simulink model "M2C_IM_CL_V1_NCADMM_Sim"  (R2023a)
settings: Solver=ode4  StartTime=0.0  StopTime=t_sim  FixedStep=tsim  RelTol=1e-3
model workspace (MAT data in the model file):
  global_can_baud_rate = '1000000'
  global_ip_addresses = {'', '', '', ''}
values from neighbouring files (symbols this model uses):
  A = [1 1 1 0 0 0 ... (first row only)    [M2C_init.m]    (also in MMCC_Sim_Script_BCD_activeset.m = -[1 0 0 1 0 0 1 0 0; 0 1 0 0 1 0 0 1 0; 0 0 1 0 0 1 0 0 1; -; MMCC_Sim_Script_BCD_activeset_LH.m = -[1 0 0 1 0 0 1 0 0; 0 1 0 0 1 0 0 1 0; 0 0 1 0 0 1 0 0 1; -)
  A11 = -(1/tau_sig)*eye(2)    [M2C_init.m]
  A21 = (Lm/tau_r)*eye(2)    [M2C_init.m]
  A_admm = zeros(2*Np, Np)    [M2C_init.m]
  A_cc = [1 0 ... (first row only)    [M2C_init.m]
  b_admm_1 = imax_admm*ones(2*Np,1)    [M2C_init.m]
  b_cc = Vmax_cc*ones(4,1)    [M2C_init.m]
  c_admm = -imax_admm*ones(Np,1)    [M2C_init.m]
  C_obs = [eye(2) zeros(2)]    [M2C_init.m]
  C_sm = 987e-6    (= 0.000987)    [M2C_init.m]
  G_cc = [1 1 ... (first row only)    [M2C_init.m]
  J_imag = [0 -1 ... (first row only)    [M2C_init.m]
  K_obsm = K_obs2'    [M2C_init.m]
  K_obsp = K_obs1'    [M2C_init.m]
  kr = Lm/Lr    (= 0.989061842659)    [M2C_init.m]
  L = 5e-3    (= 0.005)    [M2C_init.m]    (also in MMCC_Sim_Script_BCD_activeset.m = 0.02; MMCC_Sim_Script_BCD_activeset_LH.m = 0.02)
  Lsigmar = 2.6e-3    (= 0.0026)    [M2C_init.m]
  Lsigmas = 2.6e-3    (= 0.0026)    [M2C_init.m]
  N = [1/sqrt(3) 0;-1/(2*sqrt(3)) 1/2;-1/(2*sqrt(3)) -1/2;-1/sqrt(3) 0;1/(2*sqrt(3)) -1/2;1/(2*sqrt(3)) 1/2]    [M2C_init.m]    (also in MMCC_Sim_Script_BCD_activeset.m = null(A,'rational'); MMCC_Sim_Script_BCD_activeset_LH.m = [-0.4430   -0.4780    0.0994    0.0994)
  n = 4    [M2C_init.m]
  p = 2    [M2C_init.m]
  phirN = 1*Vb/ws_nom    [M2C_init.m]
  prmt_ADMM = [n, lambda_z, rho, lambda_e, C_sm, Np, imax_admm]    [M2C_init.m]
  prmt_bkpsi = [ts, Np, lambda_o, imax_admm]    [M2C_init.m]
  prmt_CCMPC = [ts, L, lambda_u, lambda_i, R, e]    [M2C_init.m]
  prmt_OBS = [ts, kr, sigma, Ls, tau_r]    [M2C_init.m]
  R = 0.2    [M2C_init.m]    (also in MMCC_Sim_Script_BCD_activeset.m = 0.001; MMCC_Sim_Script_BCD_activeset_LH.m = 0.001)
  Rr = 1.8    [M2C_init.m]
  Rs = 1.8    [M2C_init.m]
  Rsig = Rs + Rr*kr^2    (= 3.56083799149)    [M2C_init.m]
  SN = PN/FPn    (= 3703.7037037)    [M2C_init.m]
  T = [An ... (first row only)    [M2C_init.m]    (also in MMCC_Sim_Script_BCD_activeset.m = [1   0 ; -1/2  sqrt(3)/2; -1/2  -sqrt(3)/2]; MMCC_Sim_Script_BCD_activeset_LH.m = [1   0 ; -1/2  sqrt(3)/2; -1/2  -sqrt(3)/2])
  t_arranque = t_flux + 5/(dam*wn_flux) + 0.4    [M2C_init.m]
  t_flux = t_maq + 0.1    (= 0.3)    [M2C_init.m]
  t_load = t_arranque    [M2C_init.m]
  Tab0 = (1/3)*[2 -1 -1 ... (first row only)    [M2C_init.m]
  Tabc = [1 0; -.5 sqrt(3)/2; -.5 -sqrt(3)/2]    [M2C_init.m]
  tau_r = Lr/Rr    (= 0.132055555556)    [M2C_init.m]
  TN = PN/(nN*pi/30)    (= 19.7571653493)    [M2C_init.m]
  ts = 1/fs    (= 0.000166666666667)    [M2C_init.m]
  tsim = ts/40    (= 4.16666666667e-06)    [M2C_init.m]
  Vc0 = n*Vc_sm    (= 520)    [M2C_init.m]    (also in MMCC_Sim_Script_BCD_activeset.m = 18000; MMCC_Sim_Script_BCD_activeset_LH.m = 18000)
  Vc_sm = 130    [M2C_init.m]
  Vdc = n*Vc_sm    (= 520)    [M2C_init.m]
undefined symbols (not defined in the file or in its folder): Down, M2C_ADMM_Init_IM_V1, plecs, Up
libraries: spsIGBTDiodeLib x48, spsVoltageMeasurementLib x36, spsSeriesRLCBranchLib x30, spsCurrentMeasurementLib x10, eePwmGenerator x6, rtlab x3, dspstat3 x2, spsControlledVoltageSourceLib x2, spsDCVoltageSourceLib x2, opal_lib x1, dspfdesign x1, spsMeanLib x1
(part 1 of 6)
settings Model: Creator=PecLab  LastModifiedBy=matix
settings SolverCC: AlgebraicLoopSolver=TrustRegion
settings DataIOCC: SaveOutput=off  SaveTime=off  ReturnWorkspaceOutputs=off
settings OptimizationCC: BlockReduction=off  OptimizeBlockIOStorage=off  BufferReuse=off  GlobalBufferReuse=off  ExpressionFolding=off  LocalBlockOutputs=off  OptimizeDataStoreBuffers=off  BusAssignmentInplaceUpdate=off
settings DebuggingCC: UnconnectedInputMsg=warning  UnconnectedOutputMsg=warning  UnconnectedLineMsg=warning  UnderSpecifiedDimensionMsg=warning  ArithmeticOperatorsInVariantConditions=warning
settings ModelReferenceCC: EnableRefExpFcnMdlSchedulingChecks=on
settings SFSimCC: CustomCodeUndefinedFunction=UseInterfaceOnly
settings RTWCC: DLArmComputeVersion=19.05

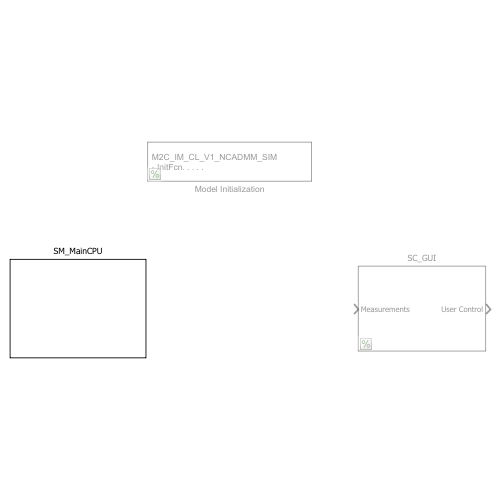
[thumbnail: Simulink's stored preview of the top-level diagram]
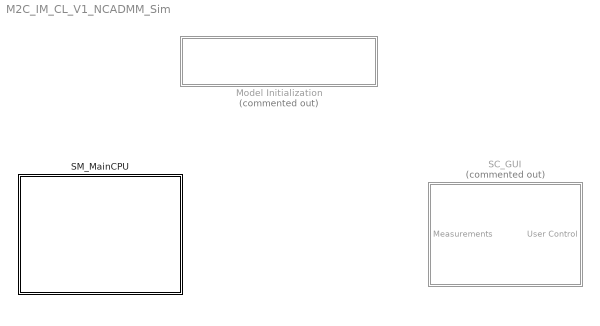
== system M2C_IM_CL_V1_NCADMM_Sim ==
  Model Initialization : Subsystem  Commented=on  mask(Model Functions){InitFcnX=, prel=off, posl=on, inif=on, strf=off}
      mask prompts: InitFcnX "Initialisation"; prel "Preload Function"; posl "PostLoad Function"; inif "InitFcn"; strf "StartFcn"
      mask init:
      | currentBlock = gcb;
      | root = bdroot(currentBlock);
      | 
      | if ~strcmp(get_param(root,'BlockDiagramType'),'library')
      |     if prel==1
      |         set_param(root, 'PreLoadFcn', InitFcnX);
      |     else
      |         set_param(root, 'PreLoadFcn', '');
      |     end
      |     if inif==1
      |         set_param(root, 'InitFcn', InitFcnX);
      |     else
      |         set_param(root, 'InitFcn', '');
      |     end
      |     if strf==1
      |         set_param(root, 'StartFcn', InitFcnX);
      |     else
      |         set_param(root, 'StartFcn', '');
      |     end
      |     if posl==1
      |         set_param(root, 'PostLoadFcn', InitFcnX);
      |     else
      |         set_param(root, 'PostLoadFcn', '');
      |     end
      | end
      | 
      | pos = get_param(currentBlock, 'Position');
      | width = pos(3) - pos(1); height = pos(4) - pos(2);
      | txt = [ upper(root) '\n' '- InitFcn. . . . . '  get_param(root, 'InitFcn') ];
      settings: CopyFcn=set_param(gcb,'LinkStatus','none')
      mask Display: text(5, height*0.5, txt, 'horizontalAlignment', 'left', 'verticalAlignment', 'middle') ;
  SC_GUI : Subsystem  Commented=on  InitFcn=M2C_ADMM_Init_IM_V1
  SM_MainCPU : Subsystem  InitFcn=M2C_ADMM_Init_IM_V1;

== system M2C_IM_CL_V1_NCADMM_Sim/Model Initialization ==

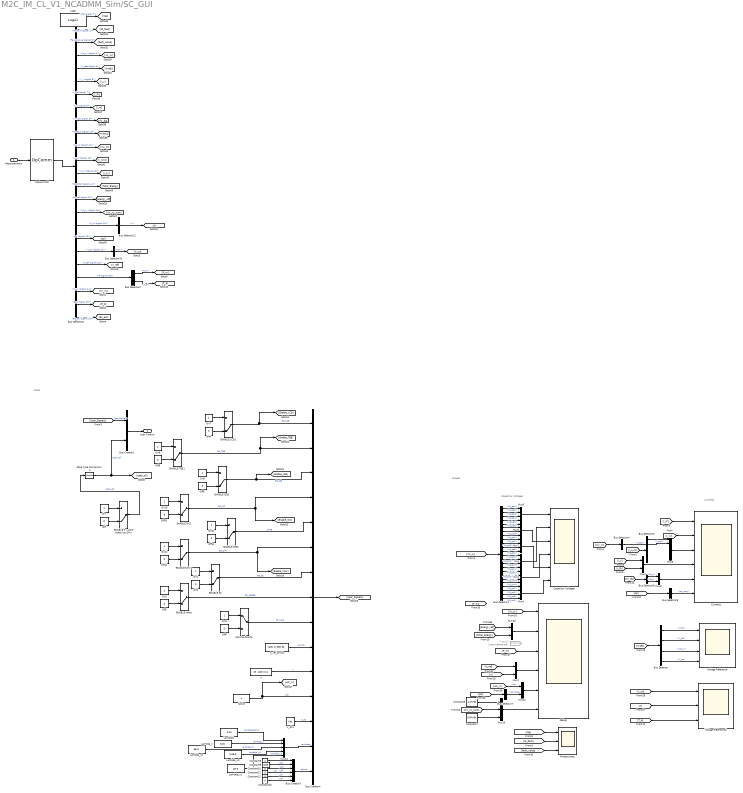
== system M2C_IM_CL_V1_NCADMM_Sim/SC_GUI ==
  note: Capacitor Voltages
  note: Panel
  note: Scopes
  note: Currents
  Measurements : Inport
  Bus Creator1 : BusCreator  Inputs=2
  Bus Creator3 : BusCreator  Inputs=6
  Bus Creator4 : BusCreator  Inputs=15
  Bus Selector : BusSelector  OutputSignals=V_s0,V_sPr,Vsm_r,V_se
  Bus Selector1 : BusSelector  OutputSignals=Vc_ap.Vc_ap1,Vc_ap.Vc_ap2,Vc_ap.Vc_ap3,Vc_ap.Vc_ap4,Vc_bp.Vc_bp1,Vc_bp.Vc_bp2,Vc_bp.Vc_bp3,Vc_bp.Vc_bp4,Vc_cp.Vc_cp1,Vc_cp.Vc_cp2,Vc_cp.Vc_cp3,Vc_cp.Vc_cp4,Vc_an.Vc_an1,Vc_an.Vc_an2,Vc_an.Vc_an3,Vc_an.Vc_an4,Vc_bn.Vc_bn1,Vc_bn.Vc_bn2,Vc_bn.Vc_bn3,Vc_bn.Vc_bn4,Vc_cn.Vc_cn1,Vc_cn.Vc_cn2,Vc_cn.Vc_cn3,Vc_cn.Vc_cn4
  Bus Selector10 : BusSelector  OutputSignals=Vcn
  Bus Selector11 : BusSelector  OutputSignals=n
  Bus Selector2 : BusSelector  OutputSignals=P_m,T_e
  Bus Selector4 : BusSelector  OutputSignals=i_apzr
  Bus Selector5 : BusSelector  OutputSignals=i_apz,i_bpz,i_cpz,i_anz,i_bnz,i_cnz
  Bus Selector6 : BusSelector  OutputSignals=log (signal 1),ID_fault (signal 2),Fault_value (signal 3),Vc_xy (signal 4),V_refs (signal 5),i_y (signal 6),i_dcr (signal 7),i_x (signal 8),im_dq (signal 9),theta_s (signal 10),i_xyzr (signal 11),i_xyz (signal 12),i_xy (signal 13),En_total (signal 14),En_ref (signal 15),Vc_xy (signal 16),n_m (signal 18),psi (signal 20),V_cn (signal 21),n_ref (signal 22),P (signal 23),Vr_xy (signal 24),E_p (signal 25),EN_ext (signal 26)
  Bus Selector7 : BusSelector  OutputSignals=psi_mag
  Bus Selector8 : BusSelector  OutputSignals=psi_ang
  Bus Selector9 : BusSelector  OutputSignals=idq_r,idq
  Capacitor Voltages : Scope  NumInputPorts=6
  Constant{10..13} (4 alike) : Constant  Value=0
  Constant6 : Constant  Value=1.1*Vdc
  Constant7 : Constant  Value=0.9*Vdc
  Constant8 : Constant
  Constant9 : Constant  Value=3.65
  Currents : Scope  NumInputPorts=6
  Data Type Conversion2 : DataTypeConversion  OutDataTypeStr=double  SaturateOnIntegerOverflow=off  RndMeth=Floor
  Debug : Scope  NumInputPorts=6
  ENABLE 0->Abre todos los SM's : ManualSwitch  CurrentSetting=0
  ENABLE CMV1 : ManualSwitch  CurrentSetting=0
  ENABLE ICB1 : ManualSwitch  CurrentSetting=0
  ENABLE ICB3 : ManualSwitch  CurrentSetting=0
  ENABLE LCB1 : ManualSwitch  CurrentSetting=0
  ENABLE OC1 : ManualSwitch  CurrentSetting=0
  ENABLE SC : ManualSwitch  CurrentSetting=0
  ENABLE TEB1 : ManualSwitch  CurrentSetting=0
  ENABLE ramp : ManualSwitch  CurrentSetting=0
  From14 : From  Commented=on  GotoTag=Theta_s
  Lambda1 : Constant  Value=0.04
  Lambda_cc : Constant  Value=5e-3
  Lambda_v0 : Constant  Value=0.2e-3
  Lambda_vz : Constant  Value=2e-3
  Lambda_z : Constant  Value=0.15
  Logo : opal_lib/Logo1  vide=[]
  Marcha directa : ManualSwitch
  Mux{,3..7} (6 alike) : Mux
  Mux{1..2,10..11} (4 alike) : Mux  Inputs=2
  Mux13 : Mux  Inputs=[1 6 1]
  Mux14 : Mux  Inputs=5
  Mux8 : Mux  Inputs=6
  Mux9 : Mux  Inputs=[2 2]
  Off{,1..3,7..12} (10 alike) : Constant  Value=0
  On{,1..3,7..12} (10 alike) : Constant
  OpCommSC : rtlab/OpComm  nbport=1  groupe_acq=1  subsys_rate=0  st=0  Synchronization=off  Interpolation=off  Threshold=1.0  Missed_Data=off  Sim_Time=off  Samples=off  dynSigOut=off  from_console=0  warning_done=off  writeOpCommFile=off  Offset=off
  Protecciones : Scope  NumInputPorts=3
  V_dc1 : Constant  Value=Vdc
  Voltage Reference : Scope  NumInputPorts=4
  Voltage Reference1 : Scope  NumInputPorts=3
  factor : Constant
  n : Constant  Value=[0 ; 440; 0.1]
  n_ref_prmts : Constant  Value=[400, 0, 300, 6]
  User Control : Outport  VectorParamsAs1DForOutWhenUnconnected=off
  wires:
  Measurements/1 -> OpCommSC/1
  Bus Creator1/1 -> User Control/1
  [Vc_xy] -> Bus Selector1/1
  Mux5/1 -> Capacitor Voltages/1
  Off/1 -> ENABLE 0->Abre todos los SM's/2
  On/1 -> ENABLE 0->Abre todos los SM's/1
  ENABLE 0->Abre todos los SM's/1 -> Data Type Conversion2/1  "open_all"
  Data Type Conversion2/1 -> Bus Creator1/2, [open_all]  "open_all"
  Mux/1 -> Capacitor Voltages/2
  Mux6/1 -> Capacitor Voltages/3
  Mux3/1 -> Capacitor Voltages/4
  Mux7/1 -> Capacitor Voltages/5
  Mux4/1 -> Capacitor Voltages/6
  [User_Signals] -> Bus Creator1/1  "User_Signals"
  Bus Selector1/1 -> Mux5/1  "<Vc_ap1>"
  Bus Selector1/2 -> Mux5/2  "<Vc_ap2>"
  Bus Selector1/3 -> Mux5/3  "<Vc_ap3>"
  Bus Selector1/4 -> Mux5/4  "<Vc_ap4>"
  Bus Selector1/5 -> Mux6/1  "<Vc_bp1>"
  Bus Selector1/6 -> Mux6/2  "<Vc_bp2>"
  Bus Selector1/7 -> Mux6/3  "<Vc_bp3>"
  Bus Selector1/8 -> Mux6/4  "<Vc_bp4>"
  Bus Selector1/9 -> Mux7/1  "<Vc_cp1>"
  Bus Selector1/10 -> Mux7/2  "<Vc_cp2>"
  Bus Selector1/11 -> Mux7/3  "<Vc_cp3>"
  Bus Selector1/12 -> Mux7/4  "<Vc_cp4>"
  Bus Selector1/13 -> Mux/1  "<Vc_an1>"
  Bus Selector1/14 -> Mux/2  "<Vc_an2>"
  Bus Selector1/15 -> Mux/3  "<Vc_an3>"
  Bus Selector1/16 -> Mux/4  "<Vc_an4>"
  Bus Selector1/17 -> Mux3/1  "<Vc_bn1>"
  Bus Selector1/18 -> Mux3/2  "<Vc_bn2>"
  Bus Selector1/19 -> Mux3/3  "<Vc_bn3>"
  Bus Selector1/20 -> Mux3/4  "<Vc_bn4>"
  Bus Selector1/21 -> Mux4/1  "<Vc_cn1>"
  Bus Selector1/22 -> Mux4/2  "<Vc_cn2>"
  Bus Selector1/23 -> Mux4/3  "<Vc_cn3>"
  Bus Selector1/24 -> Mux4/4  "<Vc_cn4>"
  [Vrefs] -> Bus Selector/1
  Bus Selector/1 -> Voltage Reference/1  "<V_s0>"
  Bus Selector/2 -> Voltage Reference/2  "<V_sPr>"
  Bus Selector/3 -> Voltage Reference/3  "<Vsm_r>"
  Bus Selector/4 -> Voltage Reference/4  "<V_se>"
  [fault_value] -> Protecciones/3
  [log] -> Protecciones/1
  [ID_fault] -> Protecciones/2
  Bus Creator4/1 -> [User_Signals]
  Off7/1 -> ENABLE LCB1/2
  Off10/1 -> ENABLE OC1/2
  On8/1 -> ENABLE TEB1/1
  On11/1 -> ENABLE ICB3/1
  Lambda_cc/1 -> Mux14/3  "lambda_cc"
  On7/1 -> ENABLE LCB1/1
  Constant12/1 -> Bus Creator3/5  "i_bn"
  Lambda1/1 -> Mux14/1  "lambda_admm"
  ENABLE LCB1/1 -> [Enable_LCB], Bus Creator4/1  "EN_LCB"
  On12/1 -> ENABLE CMV1/1
  Off12/1 -> ENABLE CMV1/2
  ENABLE ICB3/1 -> Bus Creator4/5  "SAVE"
  Constant13/1 -> Bus Creator3/6  "i_cn"
  Constant8/1 -> Bus Creator3/1  "i_ap"
  Constant9/1 -> Bus Creator3/2  "i_bp"
  Constant10/1 -> Bus Creator3/3  "i_cp"
  ENABLE TEB1/1 -> [Enable_TEB], Bus Creator4/2  "EN_TEB"
  Off9/1 -> ENABLE ICB1/2
  On10/1 -> ENABLE OC1/1
  ENABLE ICB1/1 -> [Enable_ICB], Bus Creator4/3  "EN_ICB"
  Off11/1 -> ENABLE ICB3/2
  On9/1 -> ENABLE ICB1/1
  ENABLE OC1/1 -> [Enable_OC], Bus Creator4/4  "EN_OC"
  ENABLE CMV1/1 -> [Enable_CMV], Bus Creator4/6  "EN_CMV"
  Off8/1 -> ENABLE TEB1/2
  Constant11/1 -> Bus Creator3/4  "i_an"
  [i_m] -> Currents/1
  Mux8/1 -> Currents/3
  [i_y] -> Mux2/1
  [i_xy] -> Currents/2
  Mux9/1 -> Currents/5
  [i_xycc] -> Bus Selector5/1
  [ixy_zr] -> Bus Selector4/1
  [i_Pr] -> Mux2/2
  Mux2/1 -> Currents/4
  Mux10/1 -> Debug/2
  [n_ref] -> Mux1/1
  [Vc_xy_sum] -> Mux13/2
  [Total_Energy] -> Mux10/2
  Mux13/1 -> Debug/6
  Constant7/1 -> Mux13/3
  Constant6/1 -> Mux13/1
  [n] -> Mux1/2
  Mux1/1 -> Debug/4
  [Energy_ref] -> Mux10/1
  Bus Selector6/16 -> [Vc_xy_sum]  "<Vc_xy (signal 16)>"
  Bus Selector6/3 -> [fault_value]  "<Fault_value (signal 3)>"
  Bus Selector6/12 -> [i_xycc]  "<i_xyz (signal 12)>"
  Bus Selector6/15 -> [Energy_ref]  "<En_ref (signal 15)>"
  Bus Selector6/1 -> [log]  "<log (signal 1)>"
  Bus Selector6/14 -> [Total_Energy]  "<En_total (signal 14)>"
  Bus Selector6/13 -> [i_xy]  "<i_xy (signal 13)>"
  Bus Selector6/9 -> [im_dq]  "<im_dq (signal 9)>"
  Bus Selector6/10 -> [Theta_s]  "<theta_s (signal 10)>"
  Bus Selector6/11 -> [ixy_zr]  "<i_xyzr (signal 11)>"
  Bus Selector6/6 -> [i_y]  "<i_y (signal 6)>"
  Bus Selector6/2 -> [ID_fault]  "<ID_fault (signal 2)>"
  Bus Selector6/5 -> [Vrefs]  "<V_refs (signal 5)>"
  Bus Selector6/8 -> [i_m]  "<i_x (signal 8)>"
  Bus Selector6/7 -> [i_Pr]  "<i_dcr (signal 7)>"
  Bus Selector6/4 -> [Vc_xy]  "<Vc_xy (signal 4)>"
  OpCommSC/1 -> Bus Selector6/1
  Bus Selector6/18 -> [psi]  "<psi (signal 20)>"
  [psi] -> Bus Selector7/1
  [psi] -> Bus Selector8/1
  Bus Selector8/1 -> Currents/6  "<psi_ang>"
  factor/1 -> Bus Creator4/12, [psi_rr]  "psir"
  Mux11/1 -> Debug/5
  [psi_rr] -> Mux11/1  "psir"
  Bus Selector7/1 -> Mux11/2  "<psi_mag>"
  [im_dq] -> Bus Selector9/1
  Bus Selector9/1 -> Mux9/1  "<idq_r>"
  Bus Selector9/2 -> Mux9/2  "<idq>"
  Bus Selector5/1 -> Mux8/1  "<i_apz>"
  Off1/1 -> ENABLE SC/2
  On1/1 -> ENABLE SC/1
  Marcha directa/1 -> Bus Creator4/9  "Forward"
  On3/1 -> Marcha directa/1
  Off3/1 -> Marcha directa/2
  On2/1 -> ENABLE ramp/1
  ENABLE ramp/1 -> Bus Creator4/8  "EN_SPEED"
  Off2/1 -> ENABLE ramp/2
  ENABLE SC/1 -> Bus Creator4/7  "EN_SC"
  n_ref_prmts/1 -> Bus Creator4/10  "n_t_max"
  Bus Selector6/20 -> [n_ref]  "<n_ref (signal 22)>"
  Bus Selector6/19 -> Bus Selector10/1  "<V_cn (signal 21)>"
  Bus Selector10/1 -> [V_cn]  "<Vcn>"
  [V_cn] -> Voltage Reference1/1
  Bus Selector6/17 -> Bus Selector11/1  "<n_m (signal 18)>"
  Bus Selector11/1 -> [n]  "<n>"
  [n] -> Voltage Reference1/2
  Bus Selector4/1 -> Mux8/2  "<i_apzr>"
  Bus Selector6/21 -> Bus Selector2/1  "<P (signal 23)>"
  Bus Selector2/1 -> [P_m]  "<P_m>"
  Bus Selector2/2 -> [T_e]  "<T_e>"
  Bus Creator3/1 -> Bus Creator4/15  "adjust"
  Mux14/1 -> Bus Creator4/14  "lambdas"
  V_dc1/1 -> Bus Creator4/13  "V_dc"
  n/1 -> Bus Creator4/11  "n"
  Bus Selector6/22 -> [Vr_xy]  "<Vr_xy (signal 24)>"
  [Vr_xy] -> Debug/1
  Bus Selector6/23 -> [E_p]  "<E_p (signal 25)>"
  [P_m] -> Debug/3
  Bus Selector6/24 -> [En_ext]  "<EN_ext (signal 26)>"
  [T_e] -> Voltage Reference1/3
  Lambda_v0/1 -> Mux14/4  "lambda_v0"
  Lambda_z/1 -> Mux14/2  "lambda_z"
  Lambda_vz/1 -> Mux14/5  "lambda_vz"
